simulink model "DEF_IEEE14_case1_phi"  (R2022b)
settings: Solver=FixedStepAuto  StartTime=0  StopTime=10  FixedStep=Ts  RelTol=1e-3
values from neighbouring files (symbols this model uses):
  freq_sel = imag(Mode_Hz)    [Mode_Right_Eig.m]
  Mode_Rad = D(ModeSel, ModeSel)    [Mode_Right_Eig.m]
undefined symbols (not defined in the file or in its folder): ApparatusDiscreDamping, ApparatusPara, ApparatusPowerFlow, ApparatusType, Fbase, OtherInputs, Sbase, Ts, Vbase, Wbase, x_e, Ybase, Zbase
libraries: spsGroundLib x22, SimplusGT x22, spsThreePhaseSeriesRLCBranchLib x20, eeGeneralControl x18, spsThreePhaseParallelRLCBranchLib x14, spsPLLLib x4, spsThreePhaseTransformerTwoWindingsLib x3, spsFourierLib x2, spspowerguiLib x1
settings Model: Creator=y_zhu  LastModifiedBy=y_zhu

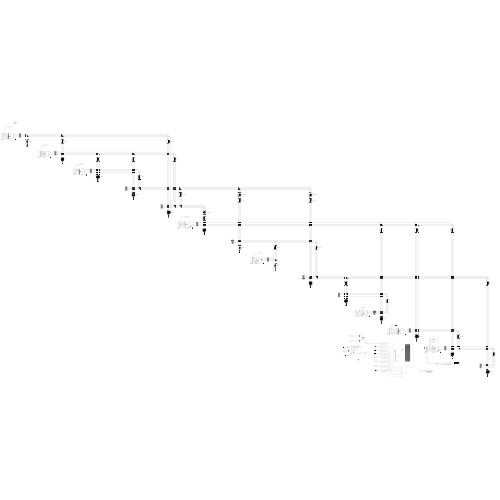
[thumbnail: Simulink's stored preview of the top-level diagram]
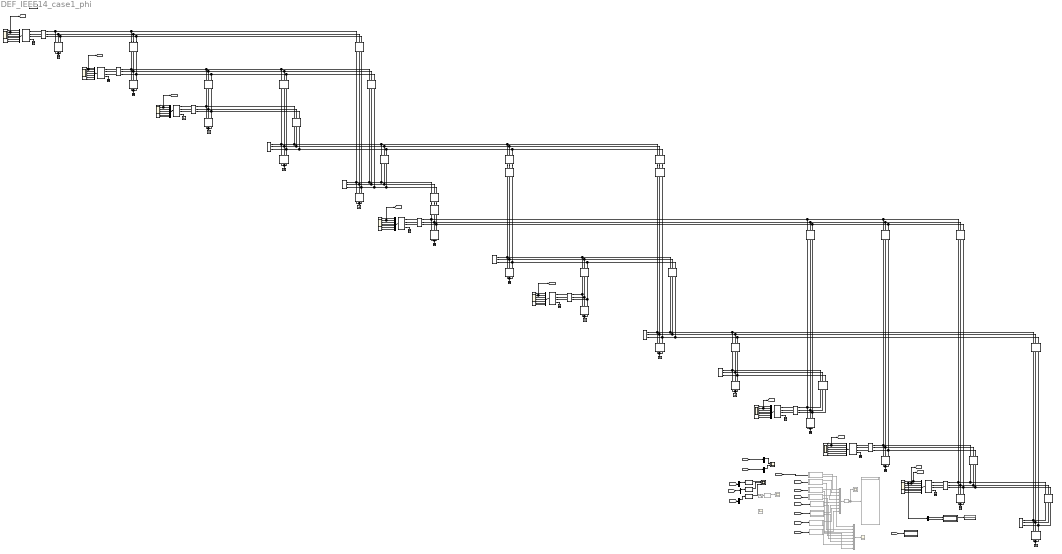
== system DEF_IEEE14_case1_phi ==
  Abs1 : Abs  Commented=on  SaturateOnIntegerOverflow=off
  B-GND{1,4,8,10,14,16,20,23..24,27,29..30,32,34} (14 alike) : spsGroundLib/Ground  LConnTagsString=a
  Branch1-1 : spsThreePhaseParallelRLCBranchLib/Three-Phase Parallel RLC Branch  LConnTagsString=A|B|C  RConnTagsString=A|B|C  BranchType=C  Resistance=(Inf)*Zbase  Inductance=(Inf)*Zbase/Wbase  Capacitance=(0.051)*Ybase/Wbase  Measurements=None
  Branch1-2 : spsThreePhaseSeriesRLCBranchLib/Three-Phase Series RLC Branch  LConnTagsString=A|B|C  RConnTagsString=A|B|C  BranchType=RL  Resistance=(0.01938)*Zbase  Inductance=(0.05917)*Zbase/Wbase  Capacitance=1e-6  Measurements=None
  Branch1-5 : spsThreePhaseSeriesRLCBranchLib/Three-Phase Series RLC Branch  LConnTagsString=A|B|C  RConnTagsString=A|B|C  BranchType=RL  Resistance=(0.05403)*Zbase  Inductance=(0.22304)*Zbase/Wbase  Capacitance=1e-6  Measurements=None
  Branch10-10 : spsThreePhaseParallelRLCBranchLib/Three-Phase Parallel RLC Branch  LConnTagsString=A|B|C  RConnTagsString=A|B|C  BranchType=RLC  Resistance=(12.2907)*Zbase  Inductance=(19.0718)*Zbase/Wbase  Capacitance=(1e-07)*Ybase/Wbase  Measurements=None
  Branch10-11 : spsThreePhaseSeriesRLCBranchLib/Three-Phase Series RLC Branch  LConnTagsString=A|B|C  RConnTagsString=A|B|C  BranchType=RL  Resistance=(0.08205)*Zbase  Inductance=(0.19207)*Zbase/Wbase  Capacitance=1e-6  Measurements=None
  Branch11-11 : spsThreePhaseParallelRLCBranchLib/Three-Phase Parallel RLC Branch  LConnTagsString=A|B|C  RConnTagsString=A|B|C  BranchType=RLC  Resistance=(10.675)*Zbase  Inductance=(62.2711)*Zbase/Wbase  Capacitance=(1e-07)*Ybase/Wbase  Measurements=None
  Branch12-12 : spsThreePhaseParallelRLCBranchLib/Three-Phase Parallel RLC Branch  LConnTagsString=A|B|C  RConnTagsString=A|B|C  BranchType=RLC  Resistance=(6.03)*Zbase  Inductance=(68.9685)*Zbase/Wbase  Capacitance=(1e-07)*Ybase/Wbase  Measurements=None
  Branch12-13 : spsThreePhaseSeriesRLCBranchLib/Three-Phase Series RLC Branch  LConnTagsString=A|B|C  RConnTagsString=A|B|C  BranchType=RL  Resistance=(0.22092)*Zbase  Inductance=(0.19988)*Zbase/Wbase  Capacitance=1e-6  Measurements=None
  Branch13-13 : spsThreePhaseParallelRLCBranchLib/Three-Phase Parallel RLC Branch  LConnTagsString=A|B|C  RConnTagsString=A|B|C  BranchType=RLC  Resistance=(2.6813)*Zbase  Inductance=(18.7232)*Zbase/Wbase  Capacitance=(1.5e-07)*Ybase/Wbase  Measurements=None
  Branch13-14 : spsThreePhaseSeriesRLCBranchLib/Three-Phase Series RLC Branch  LConnTagsString=A|B|C  RConnTagsString=A|B|C  BranchType=RL  Resistance=(0.17093)*Zbase  Inductance=(0.34802)*Zbase/Wbase  Capacitance=1e-6  Measurements=None
  Branch14-14 : spsThreePhaseParallelRLCBranchLib/Three-Phase Parallel RLC Branch  LConnTagsString=A|B|C  RConnTagsString=A|B|C  BranchType=RLC  Resistance=(7.1477)*Zbase  Inductance=(21.3001)*Zbase/Wbase  Capacitance=(1e-07)*Ybase/Wbase  Measurements=None
  Branch2-2 : spsThreePhaseParallelRLCBranchLib/Three-Phase Parallel RLC Branch  LConnTagsString=A|B|C  RConnTagsString=A|B|C  BranchType=RLC  Resistance=(5.0324)*Zbase  Inductance=(8.5986)*Zbase/Wbase  Capacitance=(0.0826)*Ybase/Wbase  Measurements=None
  Branch2-3 : spsThreePhaseSeriesRLCBranchLib/Three-Phase Series RLC Branch  LConnTagsString=A|B|C  RConnTagsString=A|B|C  BranchType=RL  Resistance=(0.04699)*Zbase  Inductance=(0.19797)*Zbase/Wbase  Capacitance=1e-6  Measurements=None
  Branch2-4 : spsThreePhaseSeriesRLCBranchLib/Three-Phase Series RLC Branch  LConnTagsString=A|B|C  RConnTagsString=A|B|C  BranchType=RL  Resistance=(0.05811)*Zbase  Inductance=(0.17632)*Zbase/Wbase  Capacitance=1e-6  Measurements=None
  Branch2-5 : spsThreePhaseSeriesRLCBranchLib/Three-Phase Series RLC Branch  LConnTagsString=A|B|C  RConnTagsString=A|B|C  BranchType=RL  Resistance=(0.05695)*Zbase  Inductance=(0.17388)*Zbase/Wbase  Capacitance=1e-6  Measurements=None
  Branch3-3 : spsThreePhaseParallelRLCBranchLib/Three-Phase Parallel RLC Branch  LConnTagsString=A|B|C  RConnTagsString=A|B|C  BranchType=RLC  Resistance=(1.0829)*Zbase  Inductance=(5.3689)*Zbase/Wbase  Capacitance=(0.0283)*Ybase/Wbase  Measurements=None
  Branch3-4 : spsThreePhaseSeriesRLCBranchLib/Three-Phase Series RLC Branch  LConnTagsString=A|B|C  RConnTagsString=A|B|C  BranchType=RL  Resistance=(0.06701)*Zbase  Inductance=(0.17103)*Zbase/Wbase  Capacitance=1e-6  Measurements=None
  Branch4-4 : spsThreePhaseParallelRLCBranchLib/Three-Phase Parallel RLC Branch  LConnTagsString=A|B|C  RConnTagsString=A|B|C  BranchType=RC  Resistance=(2.1566)*Zbase  Inductance=(Inf)*Zbase/Wbase  Capacitance=(0.061233)*Ybase/Wbase  Measurements=None
  Branch4-5 : spsThreePhaseSeriesRLCBranchLib/Three-Phase Series RLC Branch  LConnTagsString=A|B|C  RConnTagsString=A|B|C  BranchType=RL  Resistance=(0.01335)*Zbase  Inductance=(0.04211)*Zbase/Wbase  Capacitance=1e-6  Measurements=None
  Branch4-7 : spsThreePhaseSeriesRLCBranchLib/Three-Phase Series RLC Branch  LConnTagsString=A|B|C  RConnTagsString=A|B|C  BranchType=RL  Resistance=(1e-07)*Zbase  Inductance=(0.20912)*Zbase/Wbase  Capacitance=1e-6  Measurements=None
  Branch4-9 : spsThreePhaseSeriesRLCBranchLib/Three-Phase Series RLC Branch  LConnTagsString=A|B|C  RConnTagsString=A|B|C  BranchType=RL  Resistance=(1e-07)*Zbase  Inductance=(0.55618)*Zbase/Wbase  Capacitance=1e-6  Measurements=None
  Branch5-5 : spsThreePhaseParallelRLCBranchLib/Three-Phase Parallel RLC Branch  LConnTagsString=A|B|C  RConnTagsString=A|B|C  BranchType=RLC  Resistance=(13.5986)*Zbase  Inductance=(64.5935)*Zbase/Wbase  Capacitance=(0.0419)*Ybase/Wbase  Measurements=None
  Branch5-6 : spsThreePhaseSeriesRLCBranchLib/Three-Phase Series RLC Branch  LConnTagsString=A|B|C  RConnTagsString=A|B|C  BranchType=RL  Resistance=(1e-07)*Zbase  Inductance=(0.25202)*Zbase/Wbase  Capacitance=1e-6  Measurements=None
  Branch6-11 : spsThreePhaseSeriesRLCBranchLib/Three-Phase Series RLC Branch  LConnTagsString=A|B|C  RConnTagsString=A|B|C  BranchType=RL  Resistance=(0.09498)*Zbase  Inductance=(0.1989)*Zbase/Wbase  Capacitance=1e-6  Measurements=None
  Branch6-12 : spsThreePhaseSeriesRLCBranchLib/Three-Phase Series RLC Branch  LConnTagsString=A|B|C  RConnTagsString=A|B|C  BranchType=RL  Resistance=(0.12291)*Zbase  Inductance=(0.25581)*Zbase/Wbase  Capacitance=1e-6  Measurements=None
  Branch6-13 : spsThreePhaseSeriesRLCBranchLib/Three-Phase Series RLC Branch  LConnTagsString=A|B|C  RConnTagsString=A|B|C  BranchType=RL  Resistance=(0.06615)*Zbase  Inductance=(0.13027)*Zbase/Wbase  Capacitance=1e-6  Measurements=None
  Branch6-6 : spsThreePhaseParallelRLCBranchLib/Three-Phase Parallel RLC Branch  LConnTagsString=A|B|C  RConnTagsString=A|B|C  BranchType=RLC  Resistance=(10.2223)*Zbase  Inductance=(15.2653)*Zbase/Wbase  Capacitance=(2e-07)*Ybase/Wbase  Measurements=None
  Branch7-7 : spsThreePhaseParallelRLCBranchLib/Three-Phase Parallel RLC Branch  LConnTagsString=A|B|C  RConnTagsString=A|B|C  BranchType=C  Resistance=(Inf)*Zbase  Inductance=(Inf)*Zbase/Wbase  Capacitance=(1.5e-07)*Ybase/Wbase  Measurements=None
  Branch7-8 : spsThreePhaseSeriesRLCBranchLib/Three-Phase Series RLC Branch  LConnTagsString=A|B|C  RConnTagsString=A|B|C  BranchType=RL  Resistance=(1e-07)*Zbase  Inductance=(0.17615)*Zbase/Wbase  Capacitance=1e-6  Measurements=None
  Branch7-9 : spsThreePhaseSeriesRLCBranchLib/Three-Phase Series RLC Branch  LConnTagsString=A|B|C  RConnTagsString=A|B|C  BranchType=RL  Resistance=(1e-07)*Zbase  Inductance=(0.11001)*Zbase/Wbase  Capacitance=1e-6  Measurements=None
  Branch8-8 : spsThreePhaseParallelRLCBranchLib/Three-Phase Parallel RLC Branch  LConnTagsString=A|B|C  RConnTagsString=A|B|C  BranchType=C  Resistance=(Inf)*Zbase  Inductance=(Inf)*Zbase/Wbase  Capacitance=(5e-08)*Ybase/Wbase  Measurements=None
  Branch9-10 : spsThreePhaseSeriesRLCBranchLib/Three-Phase Series RLC Branch  LConnTagsString=A|B|C  RConnTagsString=A|B|C  BranchType=RL  Resistance=(0.03181)*Zbase  Inductance=(0.0845)*Zbase/Wbase  Capacitance=1e-6  Measurements=None
  Branch9-14 : spsThreePhaseSeriesRLCBranchLib/Three-Phase Series RLC Branch  LConnTagsString=A|B|C  RConnTagsString=A|B|C  BranchType=RL  Resistance=(0.12711)*Zbase  Inductance=(0.27038)*Zbase/Wbase  Capacitance=1e-6  Measurements=None
  Branch9-9 : spsThreePhaseParallelRLCBranchLib/Three-Phase Parallel RLC Branch  LConnTagsString=A|B|C  RConnTagsString=A|B|C  BranchType=RLC  Resistance=(3.7813)*Zbase  Inductance=(6.7198)*Zbase/Wbase  Capacitance=(0.19)*Ybase/Wbase  Measurements=None
  Bus Creator : BusCreator  Commented=on  Inputs=8
  Bus{1..14} (14 alike) : SimplusGT/Three-Phase Bus  Vbase=1  Sbase=1
      settings: SourceProductName=Simplus Grid Tool
  D-GND{1..3,6,8,11..13} (8 alike) : spsGroundLib/Ground  LConnTagsString=a
  D-Scope{1..3,6,8,11..13} (8 alike) : Scope  NumInputPorts=7
  DS-Bus{1..3,6,8,11..13} (8 alike) : BusSelector  OutputSignals=v_dq,i_dq,v_abc,i_abc,w,theta,pq
  Demux{,1..5} (6 alike) : Demux  Outputs=2
  Display : Display
  Display1 : Display  Commented=on
  Mux : Mux  Commented=on  Inputs=8
  PLL : spsPLLLib/PLL  Commented=on  Fmin=freq_sel/2  Par_Init=[0, 0.1]  ParK=[2.4, 1.52*10, 0]  TcD=1  MaxRateChangeFreq=1  FilterCutOffFreq=freq_sel  Ts=1/50  AGC=off
      settings: LibrarySourceBlock=sps_lib/Control/PLL
  PLL1 : spsPLLLib/PLL  Fmin=freq_sel/2  Par_Init=[0, freq_sel]  ParK=[18, 100, 1]  TcD=4e-2  MaxRateChangeFreq=1  FilterCutOffFreq=4  Ts=1e-2  AGC=on
      settings: LibrarySourceBlock=sps_lib/Control/PLL
  PLL2 : spsPLLLib/PLL  Fmin=freq_sel/2  Par_Init=[0, freq_sel]  ParK=[18, 100, 1]  TcD=4e-2  MaxRateChangeFreq=1  FilterCutOffFreq=4  Ts=1e-2  AGC=on
      settings: LibrarySourceBlock=sps_lib/Control/PLL
  PLL3 : spsPLLLib/PLL  Fmin=freq_sel/2  Par_Init=[0, freq_sel]  ParK=[18, 100, 1]  TcD=4e-2  MaxRateChangeFreq=1  FilterCutOffFreq=4  Ts=1e-2  AGC=on
      settings: LibrarySourceBlock=sps_lib/Control/PLL
  SM1 : SimplusGT/SynchronousMachineFull_Cyp_SMAVRPSSGOV (dq-Frame System Object)  Ts=Ts  Sbase=Sbase  Vbase=Vbase  Wbase=Wbase  ApparatusType=ApparatusType{1}  ApparatusPara=ApparatusPara{1}  PowerFlow=ApparatusPowerFlow{1}  x0=x_e{1}  OtherInputs=OtherInputs{1}  DiscreMethod=Hybrid Trapezoidal  EnableInsideModification=off  DiscreDampingFlag=on  DiscreDampingValue=ApparatusDiscreDamping{1}  LinearizationTimes=1  DirectFeedthrough=off
      settings: SourceProductName=Simplus Grid Tool
  SM2 : SimplusGT/SynchronousMachineFull_Cyp_SMAVRPSSGOV (dq-Frame System Object)  Ts=Ts  Sbase=Sbase  Vbase=Vbase  Wbase=Wbase  ApparatusType=ApparatusType{2}  ApparatusPara=ApparatusPara{2}  PowerFlow=ApparatusPowerFlow{2}  x0=x_e{2}  OtherInputs=OtherInputs{2}  DiscreMethod=Hybrid Trapezoidal  EnableInsideModification=off  DiscreDampingFlag=on  DiscreDampingValue=ApparatusDiscreDamping{2}  LinearizationTimes=1  DirectFeedthrough=off
      settings: SourceProductName=Simplus Grid Tool
  SM3 : SimplusGT/SynchronousMachineFull_Cyp_SMAVR (dq-Frame System Object)  Ts=Ts  Sbase=Sbase  Vbase=Vbase  Wbase=Wbase  ApparatusType=ApparatusType{3}  ApparatusPara=ApparatusPara{3}  PowerFlow=ApparatusPowerFlow{3}  x0=x_e{3}  OtherInputs=OtherInputs{3}  DiscreMethod=Hybrid Trapezoidal  EnableInsideModification=off  DiscreDampingFlag=on  DiscreDampingValue=ApparatusDiscreDamping{3}  LinearizationTimes=1  DirectFeedthrough=off
      settings: SourceProductName=Simplus Grid Tool
  SM6 : SimplusGT/SynchronousMachineFull_Cyp_SMAVR (dq-Frame System Object)  Ts=Ts  Sbase=Sbase  Vbase=Vbase  Wbase=Wbase  ApparatusType=ApparatusType{6}  ApparatusPara=ApparatusPara{6}  PowerFlow=ApparatusPowerFlow{6}  x0=x_e{6}  OtherInputs=OtherInputs{6}  DiscreMethod=Hybrid Trapezoidal  EnableInsideModification=off  DiscreDampingFlag=on  DiscreDampingValue=ApparatusDiscreDamping{6}  LinearizationTimes=1  DirectFeedthrough=off
      settings: SourceProductName=Simplus Grid Tool
  SM8 : SimplusGT/SynchronousMachineFull_Cyp_SMAVR (dq-Frame System Object)  Ts=Ts  Sbase=Sbase  Vbase=Vbase  Wbase=Wbase  ApparatusType=ApparatusType{8}  ApparatusPara=ApparatusPara{8}  PowerFlow=ApparatusPowerFlow{8}  x0=x_e{8}  OtherInputs=OtherInputs{8}  DiscreMethod=Hybrid Trapezoidal  EnableInsideModification=off  DiscreDampingFlag=on  DiscreDampingValue=ApparatusDiscreDamping{8}  LinearizationTimes=1  DirectFeedthrough=off
      settings: SourceProductName=Simplus Grid Tool
  SSO_analysis1 : Subsystem  Commented=on
  SSO_analysis2 : Subsystem  Commented=on
  SSO_analysis3 : Subsystem  Commented=on
  SSO_analysis4 : Subsystem  Commented=on
  SSO_analysis5 : Subsystem  Commented=on
  SSO_analysis6 : Subsystem  Commented=on
  SSO_analysis7 : Subsystem  Commented=on
  SSO_analysis8 : Subsystem  Commented=on
  SSO_analysis9 : Subsystem
  Scope : Scope  NumInputPorts=2
  Scope{1..3,5} (4 alike) : Scope  Commented=on
  Scope4 : Scope  NumInputPorts=3
  Sine Wave : Sin  Commented=on  Frequency=freq_sel*2*pi  SampleTime=0
  Subsystem : Subsystem
  Transformer4-7 : spsThreePhaseTransformerTwoWindingsLib/Three-Phase Transformer (Two Windings)  Winding1Connection=Yg  Winding2Connection=Yg  CoreType=Three single-phase transformers  SetSaturation=off  Hysteresis=off  DataFile='hysteresis'  SetInitialFlux=off  Measurements=None  UNITS=pu  NominalPower=[Sbase, Fbase]  Winding1=[0.978*Vbase, 0, 0]  Winding2=[Vbase, 0, 0]  Rm=1e4  Lm=1e4  L0=0.5  Saturation=[ 0,0 ; 0.0024,1.2 ; 1.0,1.52 ]  InitialFluxes=[ 0.8 , -0.8 , 0.7 ]  BreakLoop=off  DiscreteSolver=Trapezoidal iterative  DataType=off  TransfoNumber=1
  Transformer4-9 : spsThreePhaseTransformerTwoWindingsLib/Three-Phase Transformer (Two Windings)  Winding1Connection=Yg  Winding2Connection=Yg  CoreType=Three single-phase transformers  SetSaturation=off  Hysteresis=off  DataFile='hysteresis'  SetInitialFlux=off  Measurements=None  UNITS=pu  NominalPower=[Sbase, Fbase]  Winding1=[0.969*Vbase, 0, 0]  Winding2=[Vbase, 0, 0]  Rm=1e4  Lm=1e4  L0=0.5  Saturation=[ 0,0 ; 0.0024,1.2 ; 1.0,1.52 ]  InitialFluxes=[ 0.8 , -0.8 , 0.7 ]  BreakLoop=off  DiscreteSolver=Trapezoidal iterative  DataType=off  TransfoNumber=1
  Transformer5-6 : spsThreePhaseTransformerTwoWindingsLib/Three-Phase Transformer (Two Windings)  Winding1Connection=Yg  Winding2Connection=Yg  CoreType=Three single-phase transformers  SetSaturation=off  Hysteresis=off  DataFile='hysteresis'  SetInitialFlux=off  Measurements=None  UNITS=pu  NominalPower=[Sbase, Fbase]  Winding1=[0.932*Vbase, 0, 0]  Winding2=[Vbase, 0, 0]  Rm=1e4  Lm=1e4  L0=0.5  Saturation=[ 0,0 ; 0.0024,1.2 ; 1.0,1.52 ]  InitialFluxes=[ 0.8 , -0.8 , 0.7 ]  BreakLoop=off  DiscreteSolver=Trapezoidal iterative  DataType=off  TransfoNumber=1
  VSI-PLL11 : SimplusGT/Grid-Following Voltage-Source Inverter (dq-Frame System Object)  Ts=Ts  Sbase=Sbase  Vbase=Vbase  Wbase=Wbase  ApparatusType=ApparatusType{11}  ApparatusPara=ApparatusPara{11}  PowerFlow=ApparatusPowerFlow{11}  x0=x_e{11}  OtherInputs=OtherInputs{11}  DiscreMethod=Hybrid Trapezoidal  EnableInsideModification=off  DiscreDampingFlag=on  DiscreDampingValue=ApparatusDiscreDamping{11}  LinearizationTimes=1  DirectFeedthrough=off
      settings: SourceProductName=Simplus Grid Tool
  VSI-PLL12 : SimplusGT/Grid-Following Voltage-Source Inverter (dq-Frame System Object)  Ts=Ts  Sbase=Sbase  Vbase=Vbase  Wbase=Wbase  ApparatusType=ApparatusType{12}  ApparatusPara=ApparatusPara{12}  PowerFlow=ApparatusPowerFlow{12}  x0=x_e{12}  OtherInputs=OtherInputs{12}  DiscreMethod=Hybrid Trapezoidal  EnableInsideModification=off  DiscreDampingFlag=on  DiscreDampingValue=ApparatusDiscreDamping{12}  LinearizationTimes=1  DirectFeedthrough=off
      settings: SourceProductName=Simplus Grid Tool
  VSI-PLL13 : SimplusGT/Grid-Following Voltage-Source Inverter (dq-Frame System Object)  Ts=Ts  Sbase=Sbase  Vbase=Vbase  Wbase=Wbase  ApparatusType=ApparatusType{13}  ApparatusPara=ApparatusPara{13}  PowerFlow=ApparatusPowerFlow{13}  x0=x_e{13}  OtherInputs=OtherInputs{13}  DiscreMethod=Hybrid Trapezoidal  EnableInsideModification=off  DiscreDampingFlag=on  DiscreDampingValue=ApparatusDiscreDamping{13}  LinearizationTimes=1  DirectFeedthrough=off
      settings: SourceProductName=Simplus Grid Tool
  powergui : spspowerguiLib/powergui  Priority=1  SimulationMode=Discrete  SampleTime=Ts  frequency=60  Iterations=50  frequencyindice=0  Pbase=100e6  ErrMax=1e-4  UnitsV=kV  UnitsW=MW  buscounter=0  FunctionMessages=off  echomessages=off  EnableUseOfTLC=off  CurrentSourceSwitches=off  DisableSnubberDevices=off  DisableRonSwitches=off  DisableVfSwitches=off  DisplayEquations=off  AutomaticDiscreteSolvers=off  SolverType=Tustin/Backward Euler (TBE)  Interpol=off  ExternalGateDelay=off  methode=off  Ts=100  x0status=blocks  SPID=on  SwTol=0  HookPort=off  NonlinearTolerance=1e-4  nMaxIteration=100  ContinueOnMaxIteration=off  RestoreLinks=warning  ResistiveCurrentMeasurement=off  Frange=[0:2:500]  Ylog=off  Xlog=on  ShowGrid=off  save=off  variable=ZData  structure=0  ZoomFFT=off  StartTime=0.0  cycles=1  DisplayStyle=1  fundamental=60  FreqAxis=off  MaxFrequency=1000  frequencyindicesteady=1  RmsSteady=1  display=off
  wires:
  SM1/1 -> DS-Bus1/1
  DS-Bus1/1 -> D-Scope1/1  "<v_dq>"
  DS-Bus1/3 -> D-Scope1/3  "<v_abc>"
  DS-Bus1/4 -> D-Scope1/4  "<i_abc>"
  DS-Bus1/5 -> D-Scope1/5  "<w>"
  DS-Bus1/6 -> D-Scope1/6  "<theta>"
  DS-Bus1/7 -> D-Scope1/7  "<pq>"
  SM2/1 -> DS-Bus2/1
  DS-Bus2/1 -> D-Scope2/1  "<v_dq>"
  DS-Bus2/3 -> D-Scope2/3  "<v_abc>"
  DS-Bus2/4 -> D-Scope2/4  "<i_abc>"
  DS-Bus2/5 -> D-Scope2/5  "<w>"
  DS-Bus2/6 -> D-Scope2/6  "<theta>"
  DS-Bus2/7 -> D-Scope2/7  "<pq>"
  SM3/1 -> DS-Bus3/1
  DS-Bus3/1 -> D-Scope3/1  "<v_dq>"
  DS-Bus3/3 -> D-Scope3/3  "<v_abc>"
  DS-Bus3/4 -> D-Scope3/4  "<i_abc>"
  DS-Bus3/5 -> D-Scope3/5  "<w>"
  DS-Bus3/6 -> D-Scope3/6  "<theta>"
  DS-Bus3/7 -> D-Scope3/7  "<pq>"
  SM6/1 -> DS-Bus6/1
  DS-Bus6/1 -> D-Scope6/1  "<v_dq>"
  DS-Bus6/2 -> [A6_idq], D-Scope6/2  "<i_dq>"
  DS-Bus6/3 -> D-Scope6/3  "<v_abc>"
  DS-Bus6/4 -> D-Scope6/4  "<i_abc>"
  DS-Bus6/5 -> D-Scope6/5  "<w>"
  DS-Bus6/6 -> D-Scope6/6  "<theta>"
  DS-Bus6/7 -> D-Scope6/7  "<pq>"
  SM8/1 -> DS-Bus8/1
  DS-Bus8/1 -> D-Scope8/1  "<v_dq>"
  DS-Bus8/3 -> D-Scope8/3  "<v_abc>"
  DS-Bus8/4 -> D-Scope8/4  "<i_abc>"
  DS-Bus8/5 -> D-Scope8/5  "<w>"
  DS-Bus8/6 -> D-Scope8/6  "<theta>"
  DS-Bus8/7 -> D-Scope8/7  "<pq>"
  VSI-PLL11/1 -> DS-Bus11/1
  DS-Bus11/1 -> D-Scope11/1  "<v_dq>"
  DS-Bus11/2 -> [A11_idq], D-Scope11/2  "<i_dq>"
  DS-Bus11/3 -> D-Scope11/3  "<v_abc>"
  DS-Bus11/4 -> D-Scope11/4  "<i_abc>"
  DS-Bus11/5 -> D-Scope11/5  "<w>"
  DS-Bus11/6 -> D-Scope11/6  "<theta>"
  DS-Bus11/7 -> D-Scope11/7  "<pq>"
  VSI-PLL12/1 -> DS-Bus12/1
  DS-Bus12/1 -> D-Scope12/1  "<v_dq>"
  DS-Bus12/2 -> [A12_idq], D-Scope12/2  "<i_dq>"
  DS-Bus12/3 -> D-Scope12/3  "<v_abc>"
  DS-Bus12/4 -> D-Scope12/4  "<i_abc>"
  DS-Bus12/5 -> D-Scope12/5  "<w>"
  DS-Bus12/6 -> D-Scope12/6  "<theta>"
  DS-Bus12/7 -> D-Scope12/7  "<pq>"
  VSI-PLL13/1 -> DS-Bus13/1
  DS-Bus13/2 -> [A13_idq], Demux1/1, D-Scope13/2  "<i_dq>"
  DS-Bus13/3 -> D-Scope13/3  "<v_abc>"
  DS-Bus13/4 -> D-Scope13/4  "<i_abc>"
  DS-Bus13/5 -> D-Scope13/5  "<w>"
  DS-Bus13/6 -> D-Scope13/6  "<theta>"
  DS-Bus13/7 -> D-Scope13/7  "<pq>"
  DS-Bus13/1 -> [A13_vdq], D-Scope13/1  "<v_dq>"
  Demux1/1 -> Subsystem/1(id)
  Subsystem/1(id_sso_mag) -> Display/1
  Demux1/2 -> Subsystem/2(iq)
  Mux/1 -> Abs1/1
  [A6_idq] -> SSO_analysis3/1(idq)
  [A11_idq] -> SSO_analysis6/1(idq)
  [A12_idq] -> SSO_analysis7/1(idq)
  [A13_idq] -> SSO_analysis8/1(idq)
  DS-Bus8/2 -> [A8_idq], D-Scope8/2  "<i_dq>"
  [A8_idq] -> SSO_analysis4/1(idq)
  DS-Bus1/2 -> [A1_idq], D-Scope1/2  "<i_dq>"
  DS-Bus2/2 -> [A2_idq], D-Scope2/2  "<i_dq>"
  [A1_idq] -> SSO_analysis5/1(idq)
  [A2_idq] -> SSO_analysis1/1(idq)
  SSO_analysis5/1(idq_sso_abs) -> Mux/1
  SSO_analysis3/1(idq_sso_abs) -> Mux/4
  SSO_analysis4/1(idq_sso_abs) -> Mux/5
  SSO_analysis6/1(idq_sso_abs) -> Mux/6
  SSO_analysis7/1(idq_sso_abs) -> Mux/7
  SSO_analysis8/1(idq_sso_abs) -> Mux/8
  DS-Bus3/2 -> [A3_idq], D-Scope3/2  "<i_dq>"
  [A3_idq] -> SSO_analysis2/1(idq)
  Abs1/1 -> Scope2/1, Display1/1
  SSO_analysis2/1(idq_sso_abs) -> Mux/3
  SSO_analysis1/1(idq_sso_abs) -> Mux/2
  SSO_analysis5/2(idq_sso_abs_sum) -> Bus Creator/1  "A1"
  SSO_analysis1/2(idq_sso_abs_sum) -> Bus Creator/2  "A2"
  SSO_analysis2/2(idq_sso_abs_sum) -> Bus Creator/3  "A3"
  SSO_analysis3/2(idq_sso_abs_sum) -> Bus Creator/4  "A6"
  SSO_analysis4/2(idq_sso_abs_sum) -> Bus Creator/5  "A8"
  SSO_analysis6/2(idq_sso_abs_sum) -> Bus Creator/6  "A11"
  SSO_analysis7/2(idq_sso_abs_sum) -> Bus Creator/7  "A12"
  SSO_analysis8/2(idq_sso_abs_sum) -> Bus Creator/8  "A13"
  Bus Creator/1 -> Scope1/1
  [A13_vdq] -> SSO_analysis9/1(idq)
  [A6_idq] -> Demux/1
  [A12_idq] -> Demux2/1
  Demux/1 -> Scope/1
  Demux2/1 -> Scope/2
  [A6_idq] -> Demux3/1
  [A13_idq] -> Demux4/1
  Sine Wave/1 -> PLL/1
  PLL/1 -> Scope3/1
  Demux3/1 -> PLL1/1
  PLL1/1 -> Scope4/1
  Demux4/1 -> PLL2/1
  PLL2/1 -> Scope4/3
  PLL3/1 -> Scope4/2
  [A12_idq] -> Demux5/1
  Demux5/1 -> PLL3/1
  connections:
  SM1/LConn4 -- D-GND1/LConn1
  SM2/LConn4 -- D-GND2/LConn1
  SM3/LConn4 -- D-GND3/LConn1
  SM6/LConn4 -- D-GND6/LConn1
  SM8/LConn4 -- D-GND8/LConn1
  VSI-PLL11/LConn4 -- D-GND11/LConn1
  VSI-PLL12/LConn4 -- D-GND12/LConn1
  VSI-PLL13/LConn4 -- D-GND13/LConn1
  Branch1-1/RConn1 -- Branch1-1/RConn2 -- Branch1-1/RConn3 -- B-GND1/LConn1
  Branch2-2/RConn1 -- Branch2-2/RConn2 -- Branch2-2/RConn3 -- B-GND4/LConn1
  Branch3-3/RConn1 -- Branch3-3/RConn2 -- Branch3-3/RConn3 -- B-GND8/LConn1
  Branch4-4/RConn1 -- Branch4-4/RConn2 -- Branch4-4/RConn3 -- B-GND10/LConn1
  Branch5-5/RConn1 -- Branch5-5/RConn2 -- Branch5-5/RConn3 -- B-GND14/LConn1
  Branch6-6/RConn1 -- Branch6-6/RConn2 -- Branch6-6/RConn3 -- B-GND16/LConn1
  Branch7-7/RConn1 -- Branch7-7/RConn2 -- Branch7-7/RConn3 -- B-GND20/LConn1
  Branch8-8/RConn1 -- Branch8-8/RConn2 -- Branch8-8/RConn3 -- B-GND23/LConn1
  Branch9-9/RConn1 -- Branch9-9/RConn2 -- Branch9-9/RConn3 -- B-GND24/LConn1
  Branch10-10/RConn1 -- Branch10-10/RConn2 -- Branch10-10/RConn3 -- B-GND27/LConn1
  Branch11-11/RConn1 -- Branch11-11/RConn2 -- Branch11-11/RConn3 -- B-GND29/LConn1
  Branch12-12/RConn1 -- Branch12-12/RConn2 -- Branch12-12/RConn3 -- B-GND30/LConn1
  Branch13-13/RConn1 -- Branch13-13/RConn2 -- Branch13-13/RConn3 -- B-GND32/LConn1
  Branch14-14/RConn1 -- Branch14-14/RConn2 -- Branch14-14/RConn3 -- B-GND34/LConn1
  Branch1-2/RConn1 -- Bus2/RConn1 -- Branch2-2/LConn1 -- Branch2-5/LConn1 -- Branch2-4/LConn1 -- Branch2-3/LConn1
  Branch1-2/RConn2 -- Bus2/RConn2 -- Branch2-2/LConn2 -- Branch2-5/LConn2 -- Branch2-4/LConn2 -- Branch2-3/LConn2
  Branch1-2/RConn3 -- Bus2/RConn3 -- Branch2-2/LConn3 -- Branch2-5/LConn3 -- Branch2-4/LConn3 -- Branch2-3/LConn3
  Branch1-2/LConn1 -- Bus1/RConn1 -- Branch1-1/LConn1 -- Branch1-5/LConn1
  Branch1-2/LConn2 -- Bus1/RConn2 -- Branch1-1/LConn2 -- Branch1-5/LConn2
  Branch1-2/LConn3 -- Bus1/RConn3 -- Branch1-1/LConn3 -- Branch1-5/LConn3
  Branch1-5/RConn1 -- Bus5/RConn1 -- Branch5-5/LConn1 -- Transformer5-6/LConn1 -- Branch4-5/RConn1 -- Branch2-5/RConn1
  Branch1-5/RConn2 -- Bus5/RConn2 -- Branch5-5/LConn2 -- Transformer5-6/LConn2 -- Branch4-5/RConn2 -- Branch2-5/RConn2
  Branch1-5/RConn3 -- Bus5/RConn3 -- Branch5-5/LConn3 -- Transformer5-6/LConn3 -- Branch4-5/RConn3 -- Branch2-5/RConn3
  Branch2-3/RConn1 -- Bus3/RConn1 -- Branch3-3/LConn1 -- Branch3-4/LConn1
  Branch2-3/RConn2 -- Bus3/RConn2 -- Branch3-3/LConn2 -- Branch3-4/LConn2
  Branch2-3/RConn3 -- Bus3/RConn3 -- Branch3-3/LConn3 -- Branch3-4/LConn3
  Branch2-4/RConn1 -- Bus4/RConn1 -- Branch4-4/LConn1 -- Transformer4-9/LConn1 -- Transformer4-7/LConn1 -- Branch4-5/LConn1 -- Branch3-4/RConn1
  Branch2-4/RConn2 -- Bus4/RConn2 -- Branch4-4/LConn2 -- Transformer4-9/LConn2 -- Transformer4-7/LConn2 -- Branch4-5/LConn2 -- Branch3-4/RConn2
  Branch2-4/RConn3 -- Bus4/RConn3 -- Branch4-4/LConn3 -- Transformer4-9/LConn3 -- Transformer4-7/LConn3 -- Branch4-5/LConn3 -- Branch3-4/RConn3
  Branch4-7/RConn1 -- Bus7/RConn1 -- Branch7-7/LConn1 -- Branch7-9/LConn1 -- Branch7-8/LConn1
  Branch4-7/RConn2 -- Bus7/RConn2 -- Branch7-7/LConn2 -- Branch7-9/LConn2 -- Branch7-8/LConn2
  Branch4-7/RConn3 -- Bus7/RConn3 -- Branch7-7/LConn3 -- Branch7-9/LConn3 -- Branch7-8/LConn3
  Transformer4-7/RConn1 -- Branch4-7/LConn1
  Transformer4-7/RConn2 -- Branch4-7/LConn2
  Transformer4-7/RConn3 -- Branch4-7/LConn3
  Branch4-9/RConn1 -- Bus9/RConn1 -- Branch9-9/LConn1 -- Branch9-14/LConn1 -- Branch9-10/LConn1 -- Branch7-9/RConn1
  Branch4-9/RConn2 -- Bus9/RConn2 -- Branch9-9/LConn2 -- Branch9-14/LConn2 -- Branch9-10/LConn2 -- Branch7-9/RConn2
  Branch4-9/RConn3 -- Bus9/RConn3 -- Branch9-9/LConn3 -- Branch9-14/LConn3 -- Branch9-10/LConn3 -- Branch7-9/RConn3
  Transformer4-9/RConn1 -- Branch4-9/LConn1
  Transformer4-9/RConn2 -- Branch4-9/LConn2
  Transformer4-9/RConn3 -- Branch4-9/LConn3
  Branch5-6/RConn1 -- Bus6/RConn1 -- Branch6-6/LConn1 -- Branch6-13/LConn1 -- Branch6-12/LConn1 -- Branch6-11/LConn1
  Branch5-6/RConn2 -- Bus6/RConn2 -- Branch6-6/LConn2 -- Branch6-13/LConn2 -- Branch6-12/LConn2 -- Branch6-11/LConn2
  Branch5-6/RConn3 -- Bus6/RConn3 -- Branch6-6/LConn3 -- Branch6-13/LConn3 -- Branch6-12/LConn3 -- Branch6-11/LConn3
  Transformer5-6/RConn1 -- Branch5-6/LConn1
  Transformer5-6/RConn2 -- Branch5-6/LConn2
  Transformer5-6/RConn3 -- Branch5-6/LConn3
  Branch6-11/RConn1 -- Bus11/RConn1 -- Branch11-11/LConn1 -- Branch10-11/RConn1
  Branch6-11/RConn2 -- Bus11/RConn2 -- Branch11-11/LConn2 -- Branch10-11/RConn2
  Branch6-11/RConn3 -- Bus11/RConn3 -- Branch11-11/LConn3 -- Branch10-11/RConn3
  Branch6-12/RConn1 -- Bus12/RConn1 -- Branch12-12/LConn1 -- Branch12-13/LConn1
  Branch6-12/RConn2 -- Bus12/RConn2 -- Branch12-12/LConn2 -- Branch12-13/LConn2
  Branch6-12/RConn3 -- Bus12/RConn3 -- Branch12-12/LConn3 -- Branch12-13/LConn3
  Branch6-13/RConn1 -- Bus13/RConn1 -- Branch13-13/LConn1 -- Branch13-14/LConn1 -- Branch12-13/RConn1
  Branch6-13/RConn2 -- Bus13/RConn2 -- Branch13-13/LConn2 -- Branch13-14/LConn2 -- Branch12-13/RConn2
  Branch6-13/RConn3 -- Bus13/RConn3 -- Branch13-13/LConn3 -- Branch13-14/LConn3 -- Branch12-13/RConn3
  Branch7-8/RConn1 -- Bus8/RConn1 -- Branch8-8/LConn1
  Branch7-8/RConn2 -- Bus8/RConn2 -- Branch8-8/LConn2
  Branch7-8/RConn3 -- Bus8/RConn3 -- Branch8-8/LConn3
  Branch9-10/RConn1 -- Bus10/RConn1 -- Branch10-10/LConn1 -- Branch10-11/LConn1
  Branch9-10/RConn2 -- Bus10/RConn2 -- Branch10-10/LConn2 -- Branch10-11/LConn2
  Branch9-10/RConn3 -- Bus10/RConn3 -- Branch10-10/LConn3 -- Branch10-11/LConn3
  Branch9-14/RConn1 -- Bus14/RConn1 -- Branch14-14/LConn1 -- Branch13-14/RConn1
  Branch9-14/RConn2 -- Bus14/RConn2 -- Branch14-14/LConn2 -- Branch13-14/RConn2
  Branch9-14/RConn3 -- Bus14/RConn3 -- Branch14-14/LConn3 -- Branch13-14/RConn3
  SM1/LConn1 -- Bus1/LConn1
  SM1/LConn2 -- Bus1/LConn2
  SM1/LConn3 -- Bus1/LConn3
  SM2/LConn1 -- Bus2/LConn1
  SM2/LConn2 -- Bus2/LConn2
  SM2/LConn3 -- Bus2/LConn3
  SM3/LConn1 -- Bus3/LConn1
  SM3/LConn2 -- Bus3/LConn2
  SM3/LConn3 -- Bus3/LConn3
  SM6/LConn1 -- Bus6/LConn1
  SM6/LConn2 -- Bus6/LConn2
  SM6/LConn3 -- Bus6/LConn3
  SM8/LConn1 -- Bus8/LConn1
  SM8/LConn2 -- Bus8/LConn2
  SM8/LConn3 -- Bus8/LConn3
  VSI-PLL11/LConn1 -- Bus11/LConn1
  VSI-PLL11/LConn2 -- Bus11/LConn2
  VSI-PLL11/LConn3 -- Bus11/LConn3
  VSI-PLL12/LConn1 -- Bus12/LConn1
  VSI-PLL12/LConn2 -- Bus12/LConn2
  VSI-PLL12/LConn3 -- Bus12/LConn3
  VSI-PLL13/LConn1 -- Bus13/LConn1
  VSI-PLL13/LConn2 -- Bus13/LConn2
  VSI-PLL13/LConn3 -- Bus13/LConn3

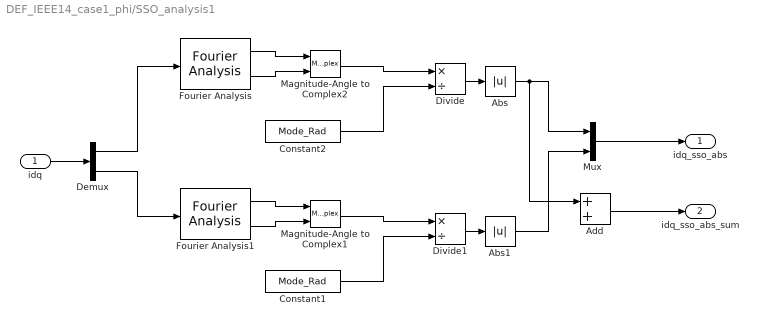
== system DEF_IEEE14_case1_phi/SSO_analysis1 ==
  idq : Inport
  Abs : Abs  SaturateOnIntegerOverflow=off
  Abs1 : Abs  SaturateOnIntegerOverflow=off
  Add : Sum
  Constant1 : Constant  Value=Mode_Rad
  Constant2 : Constant  Value=Mode_Rad
  Demux : Demux  Outputs=2
  Divide : Product  Inputs=*/
  Divide1 : Product  Inputs=*/
  Fourier Analysis : eeGeneralControl/Fourier Analysis  f=freq_sel/3  n=3  M0=0  Ph0=0  BufferSize=8192  Ts=1/50
      settings: LibrarySourceBlock=ee_sl_lib/General Control/Fourier Analysis
  Fourier Analysis1 : eeGeneralControl/Fourier Analysis  f=freq_sel/3  n=3  M0=0  Ph0=0  BufferSize=8192  Ts=1/50
      settings: LibrarySourceBlock=ee_sl_lib/General Control/Fourier Analysis
  Magnitude-Angle to Complex1 : MagnitudeAngleToComplex
  Magnitude-Angle to Complex2 : MagnitudeAngleToComplex
  Mux : Mux  Inputs=2
  idq_sso_abs : Outport
  idq_sso_abs_sum : Outport  Port=2
  wires:
  Constant2/1 -> Divide/2
  idq/1 -> Demux/1
  Demux/1 -> Fourier Analysis/1
  Fourier Analysis/1 -> Magnitude-Angle to Complex2/1
  Fourier Analysis/2 -> Magnitude-Angle to Complex2/2
  Magnitude-Angle to Complex2/1 -> Divide/1
  Mux/1 -> idq_sso_abs/1
  Divide/1 -> Abs/1
  Fourier Analysis1/2 -> Magnitude-Angle to Complex1/2
  Fourier Analysis1/1 -> Magnitude-Angle to Complex1/1
  Magnitude-Angle to Complex1/1 -> Divide1/1
  Constant1/1 -> Divide1/2
  Demux/2 -> Fourier Analysis1/1
  Divide1/1 -> Abs1/1
  Abs/1 -> Add/1, Mux/1
  Abs1/1 -> Mux/2
  Add/1 -> idq_sso_abs_sum/1

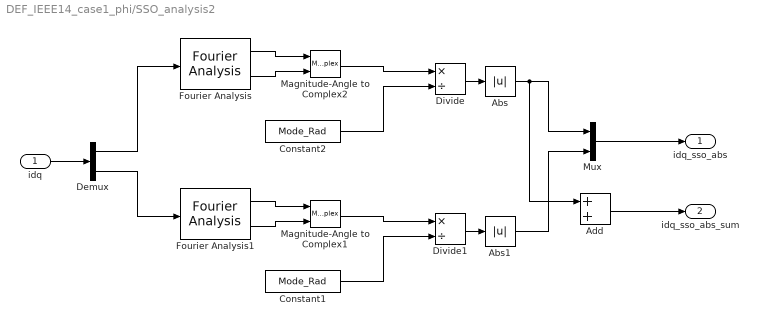
== system DEF_IEEE14_case1_phi/SSO_analysis2 ==
  idq : Inport
  Abs : Abs  SaturateOnIntegerOverflow=off
  Abs1 : Abs  SaturateOnIntegerOverflow=off
  Add : Sum
  Constant1 : Constant  Value=Mode_Rad
  Constant2 : Constant  Value=Mode_Rad
  Demux : Demux  Outputs=2
  Divide : Product  Inputs=*/
  Divide1 : Product  Inputs=*/
  Fourier Analysis : eeGeneralControl/Fourier Analysis  f=freq_sel/3  n=3  M0=0  Ph0=0  BufferSize=8192  Ts=1/50
      settings: LibrarySourceBlock=ee_sl_lib/General Control/Fourier Analysis
  Fourier Analysis1 : eeGeneralControl/Fourier Analysis  f=freq_sel/3  n=3  M0=0  Ph0=0  BufferSize=8192  Ts=1/50
      settings: LibrarySourceBlock=ee_sl_lib/General Control/Fourier Analysis
  Magnitude-Angle to Complex1 : MagnitudeAngleToComplex
  Magnitude-Angle to Complex2 : MagnitudeAngleToComplex
  Mux : Mux  Inputs=2
  idq_sso_abs : Outport
  idq_sso_abs_sum : Outport  Port=2
  wires:
  Constant2/1 -> Divide/2
  idq/1 -> Demux/1
  Demux/1 -> Fourier Analysis/1
  Fourier Analysis/1 -> Magnitude-Angle to Complex2/1
  Fourier Analysis/2 -> Magnitude-Angle to Complex2/2
  Magnitude-Angle to Complex2/1 -> Divide/1
  Mux/1 -> idq_sso_abs/1
  Divide/1 -> Abs/1
  Fourier Analysis1/2 -> Magnitude-Angle to Complex1/2
  Fourier Analysis1/1 -> Magnitude-Angle to Complex1/1
  Magnitude-Angle to Complex1/1 -> Divide1/1
  Constant1/1 -> Divide1/2
  Demux/2 -> Fourier Analysis1/1
  Divide1/1 -> Abs1/1
  Abs/1 -> Add/1, Mux/1
  Abs1/1 -> Mux/2
  Add/1 -> idq_sso_abs_sum/1

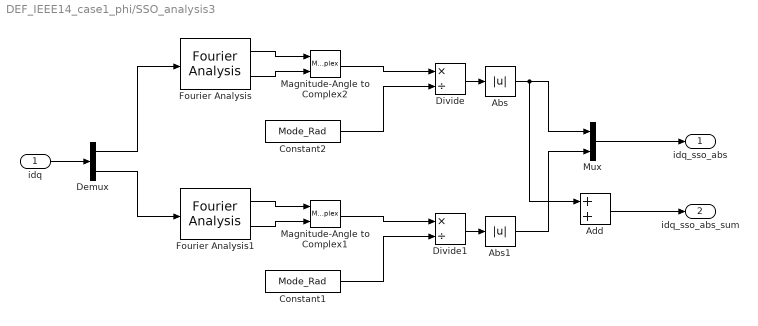
== system DEF_IEEE14_case1_phi/SSO_analysis3 ==
  idq : Inport
  Abs : Abs  SaturateOnIntegerOverflow=off
  Abs1 : Abs  SaturateOnIntegerOverflow=off
  Add : Sum
  Constant1 : Constant  Value=Mode_Rad
  Constant2 : Constant  Value=Mode_Rad
  Demux : Demux  Outputs=2
  Divide : Product  Inputs=*/
  Divide1 : Product  Inputs=*/
  Fourier Analysis : eeGeneralControl/Fourier Analysis  f=freq_sel/3  n=3  M0=0  Ph0=0  BufferSize=8192  Ts=1/50
      settings: LibrarySourceBlock=ee_sl_lib/General Control/Fourier Analysis
  Fourier Analysis1 : eeGeneralControl/Fourier Analysis  f=freq_sel/3  n=3  M0=0  Ph0=0  BufferSize=8192  Ts=1/50
      settings: LibrarySourceBlock=ee_sl_lib/General Control/Fourier Analysis
  Magnitude-Angle to Complex1 : MagnitudeAngleToComplex
  Magnitude-Angle to Complex2 : MagnitudeAngleToComplex
  Mux : Mux  Inputs=2
  idq_sso_abs : Outport
  idq_sso_abs_sum : Outport  Port=2
  wires:
  Constant2/1 -> Divide/2
  idq/1 -> Demux/1
  Demux/1 -> Fourier Analysis/1
  Fourier Analysis/1 -> Magnitude-Angle to Complex2/1
  Fourier Analysis/2 -> Magnitude-Angle to Complex2/2
  Magnitude-Angle to Complex2/1 -> Divide/1
  Mux/1 -> idq_sso_abs/1
  Divide/1 -> Abs/1
  Fourier Analysis1/2 -> Magnitude-Angle to Complex1/2
  Fourier Analysis1/1 -> Magnitude-Angle to Complex1/1
  Magnitude-Angle to Complex1/1 -> Divide1/1
  Constant1/1 -> Divide1/2
  Demux/2 -> Fourier Analysis1/1
  Divide1/1 -> Abs1/1
  Abs/1 -> Add/1, Mux/1
  Abs1/1 -> Mux/2
  Add/1 -> idq_sso_abs_sum/1

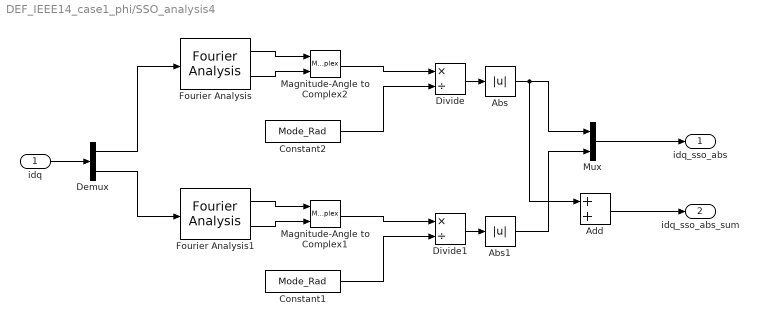
== system DEF_IEEE14_case1_phi/SSO_analysis4 ==
  idq : Inport
  Abs : Abs  SaturateOnIntegerOverflow=off
  Abs1 : Abs  SaturateOnIntegerOverflow=off
  Add : Sum
  Constant1 : Constant  Value=Mode_Rad
  Constant2 : Constant  Value=Mode_Rad
  Demux : Demux  Outputs=2
  Divide : Product  Inputs=*/
  Divide1 : Product  Inputs=*/
  Fourier Analysis : eeGeneralControl/Fourier Analysis  f=freq_sel/3  n=3  M0=0  Ph0=0  BufferSize=8192  Ts=1/50
      settings: LibrarySourceBlock=ee_sl_lib/General Control/Fourier Analysis
  Fourier Analysis1 : eeGeneralControl/Fourier Analysis  f=freq_sel/3  n=3  M0=0  Ph0=0  BufferSize=8192  Ts=1/50
      settings: LibrarySourceBlock=ee_sl_lib/General Control/Fourier Analysis
  Magnitude-Angle to Complex1 : MagnitudeAngleToComplex
  Magnitude-Angle to Complex2 : MagnitudeAngleToComplex
  Mux : Mux  Inputs=2
  idq_sso_abs : Outport
  idq_sso_abs_sum : Outport  Port=2
  wires:
  Constant2/1 -> Divide/2
  idq/1 -> Demux/1
  Demux/1 -> Fourier Analysis/1
  Fourier Analysis/1 -> Magnitude-Angle to Complex2/1
  Fourier Analysis/2 -> Magnitude-Angle to Complex2/2
  Magnitude-Angle to Complex2/1 -> Divide/1
  Mux/1 -> idq_sso_abs/1
  Divide/1 -> Abs/1
  Fourier Analysis1/2 -> Magnitude-Angle to Complex1/2
  Fourier Analysis1/1 -> Magnitude-Angle to Complex1/1
  Magnitude-Angle to Complex1/1 -> Divide1/1
  Constant1/1 -> Divide1/2
  Demux/2 -> Fourier Analysis1/1
  Divide1/1 -> Abs1/1
  Abs/1 -> Add/1, Mux/1
  Abs1/1 -> Mux/2
  Add/1 -> idq_sso_abs_sum/1

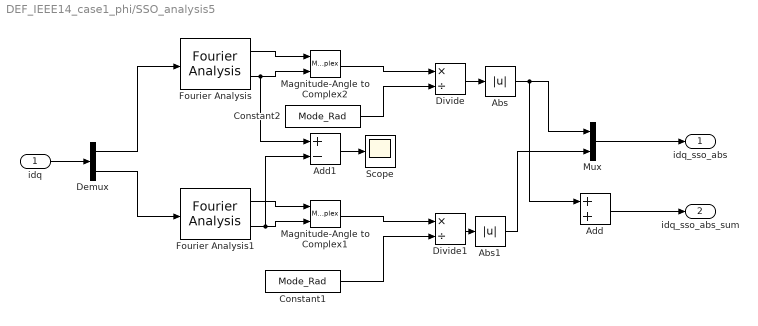
== system DEF_IEEE14_case1_phi/SSO_analysis5 ==
  idq : Inport
  Abs : Abs  SaturateOnIntegerOverflow=off
  Abs1 : Abs  SaturateOnIntegerOverflow=off
  Add : Sum
  Add1 : Sum  Inputs=+-
  Constant1 : Constant  Value=Mode_Rad
  Constant2 : Constant  Value=Mode_Rad
  Demux : Demux  Outputs=2
  Divide : Product  Inputs=*/
  Divide1 : Product  Inputs=*/
  Fourier Analysis : eeGeneralControl/Fourier Analysis  f=freq_sel/3  n=3  M0=0  Ph0=0  BufferSize=8192  Ts=1/50
      settings: LibrarySourceBlock=ee_sl_lib/General Control/Fourier Analysis
  Fourier Analysis1 : eeGeneralControl/Fourier Analysis  f=freq_sel/3  n=3  M0=0  Ph0=0  BufferSize=8192  Ts=1/50
      settings: LibrarySourceBlock=ee_sl_lib/General Control/Fourier Analysis
  Magnitude-Angle to Complex1 : MagnitudeAngleToComplex
  Magnitude-Angle to Complex2 : MagnitudeAngleToComplex
  Mux : Mux  Inputs=2
  Scope : Scope
  idq_sso_abs : Outport
  idq_sso_abs_sum : Outport  Port=2
  wires:
  Constant2/1 -> Divide/2
  idq/1 -> Demux/1
  Demux/1 -> Fourier Analysis/1
  Fourier Analysis/1 -> Magnitude-Angle to Complex2/1
  Fourier Analysis/2 -> Add1/1, Magnitude-Angle to Complex2/2
  Magnitude-Angle to Complex2/1 -> Divide/1
  Mux/1 -> idq_sso_abs/1
  Divide/1 -> Abs/1
  Fourier Analysis1/2 -> Add1/2, Magnitude-Angle to Complex1/2
  Fourier Analysis1/1 -> Magnitude-Angle to Complex1/1
  Magnitude-Angle to Complex1/1 -> Divide1/1
  Constant1/1 -> Divide1/2
  Demux/2 -> Fourier Analysis1/1
  Divide1/1 -> Abs1/1
  Abs/1 -> Add/1, Mux/1
  Abs1/1 -> Mux/2
  Add/1 -> idq_sso_abs_sum/1
  Add1/1 -> Scope/1

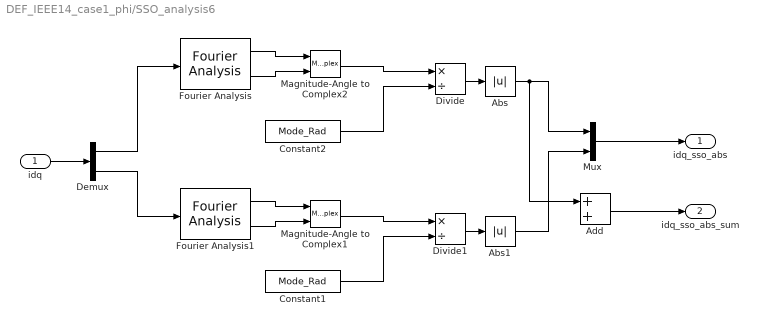
== system DEF_IEEE14_case1_phi/SSO_analysis6 ==
  idq : Inport
  Abs : Abs  SaturateOnIntegerOverflow=off
  Abs1 : Abs  SaturateOnIntegerOverflow=off
  Add : Sum
  Constant1 : Constant  Value=Mode_Rad
  Constant2 : Constant  Value=Mode_Rad
  Demux : Demux  Outputs=2
  Divide : Product  Inputs=*/
  Divide1 : Product  Inputs=*/
  Fourier Analysis : eeGeneralControl/Fourier Analysis  f=freq_sel/3  n=3  M0=0  Ph0=0  BufferSize=8192  Ts=1/50
      settings: LibrarySourceBlock=ee_sl_lib/General Control/Fourier Analysis
  Fourier Analysis1 : eeGeneralControl/Fourier Analysis  f=freq_sel/3  n=3  M0=0  Ph0=0  BufferSize=8192  Ts=1/50
      settings: LibrarySourceBlock=ee_sl_lib/General Control/Fourier Analysis
  Magnitude-Angle to Complex1 : MagnitudeAngleToComplex
  Magnitude-Angle to Complex2 : MagnitudeAngleToComplex
  Mux : Mux  Inputs=2
  idq_sso_abs : Outport
  idq_sso_abs_sum : Outport  Port=2
  wires:
  Constant2/1 -> Divide/2
  idq/1 -> Demux/1
  Demux/1 -> Fourier Analysis/1
  Fourier Analysis/1 -> Magnitude-Angle to Complex2/1
  Fourier Analysis/2 -> Magnitude-Angle to Complex2/2
  Magnitude-Angle to Complex2/1 -> Divide/1
  Mux/1 -> idq_sso_abs/1
  Divide/1 -> Abs/1
  Fourier Analysis1/2 -> Magnitude-Angle to Complex1/2
  Fourier Analysis1/1 -> Magnitude-Angle to Complex1/1
  Magnitude-Angle to Complex1/1 -> Divide1/1
  Constant1/1 -> Divide1/2
  Demux/2 -> Fourier Analysis1/1
  Divide1/1 -> Abs1/1
  Abs/1 -> Add/1, Mux/1
  Abs1/1 -> Mux/2
  Add/1 -> idq_sso_abs_sum/1

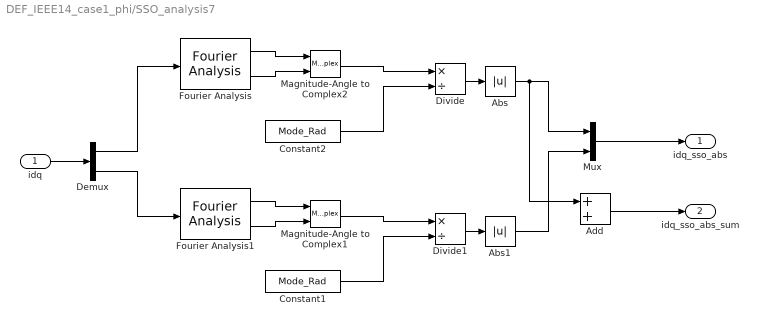
== system DEF_IEEE14_case1_phi/SSO_analysis7 ==
  idq : Inport
  Abs : Abs  SaturateOnIntegerOverflow=off
  Abs1 : Abs  SaturateOnIntegerOverflow=off
  Add : Sum
  Constant1 : Constant  Value=Mode_Rad
  Constant2 : Constant  Value=Mode_Rad
  Demux : Demux  Outputs=2
  Divide : Product  Inputs=*/
  Divide1 : Product  Inputs=*/
  Fourier Analysis : eeGeneralControl/Fourier Analysis  f=freq_sel/3  n=3  M0=0  Ph0=0  BufferSize=8192  Ts=1/50
      settings: LibrarySourceBlock=ee_sl_lib/General Control/Fourier Analysis
  Fourier Analysis1 : eeGeneralControl/Fourier Analysis  f=freq_sel/3  n=3  M0=0  Ph0=0  BufferSize=8192  Ts=1/50
      settings: LibrarySourceBlock=ee_sl_lib/General Control/Fourier Analysis
  Magnitude-Angle to Complex1 : MagnitudeAngleToComplex
  Magnitude-Angle to Complex2 : MagnitudeAngleToComplex
  Mux : Mux  Inputs=2
  idq_sso_abs : Outport
  idq_sso_abs_sum : Outport  Port=2
  wires:
  Constant2/1 -> Divide/2
  idq/1 -> Demux/1
  Demux/1 -> Fourier Analysis/1
  Fourier Analysis/1 -> Magnitude-Angle to Complex2/1
  Fourier Analysis/2 -> Magnitude-Angle to Complex2/2
  Magnitude-Angle to Complex2/1 -> Divide/1
  Mux/1 -> idq_sso_abs/1
  Divide/1 -> Abs/1
  Fourier Analysis1/2 -> Magnitude-Angle to Complex1/2
  Fourier Analysis1/1 -> Magnitude-Angle to Complex1/1
  Magnitude-Angle to Complex1/1 -> Divide1/1
  Constant1/1 -> Divide1/2
  Demux/2 -> Fourier Analysis1/1
  Divide1/1 -> Abs1/1
  Abs/1 -> Add/1, Mux/1
  Abs1/1 -> Mux/2
  Add/1 -> idq_sso_abs_sum/1

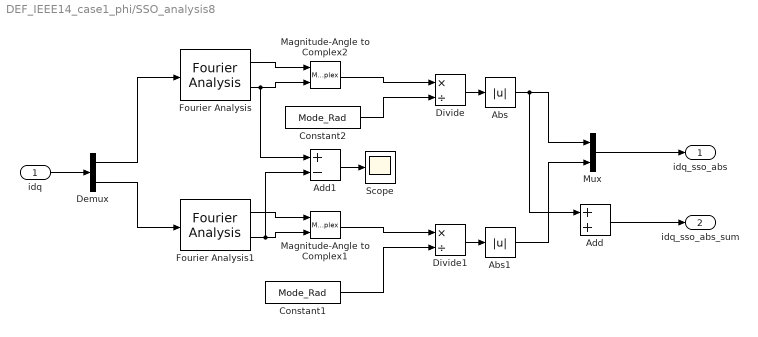
== system DEF_IEEE14_case1_phi/SSO_analysis8 ==
  idq : Inport
  Abs : Abs  SaturateOnIntegerOverflow=off
  Abs1 : Abs  SaturateOnIntegerOverflow=off
  Add : Sum
  Add1 : Sum  Inputs=+-
  Constant1 : Constant  Value=Mode_Rad
  Constant2 : Constant  Value=Mode_Rad
  Demux : Demux  Outputs=2
  Divide : Product  Inputs=*/
  Divide1 : Product  Inputs=*/
  Fourier Analysis : eeGeneralControl/Fourier Analysis  f=freq_sel/3  n=3  M0=0  Ph0=0  BufferSize=8192  Ts=1/50
      settings: LibrarySourceBlock=ee_sl_lib/General Control/Fourier Analysis
  Fourier Analysis1 : eeGeneralControl/Fourier Analysis  f=freq_sel/3  n=3  M0=0  Ph0=0  BufferSize=8192  Ts=1/50
      settings: LibrarySourceBlock=ee_sl_lib/General Control/Fourier Analysis
  Magnitude-Angle to Complex1 : MagnitudeAngleToComplex
  Magnitude-Angle to Complex2 : MagnitudeAngleToComplex
  Mux : Mux  Inputs=2
  Scope : Scope
  idq_sso_abs : Outport
  idq_sso_abs_sum : Outport  Port=2
  wires:
  Constant2/1 -> Divide/2
  idq/1 -> Demux/1
  Demux/1 -> Fourier Analysis/1
  Fourier Analysis/1 -> Magnitude-Angle to Complex2/1
  Magnitude-Angle to Complex2/1 -> Divide/1
  Mux/1 -> idq_sso_abs/1
  Divide/1 -> Abs/1
  Fourier Analysis1/1 -> Magnitude-Angle to Complex1/1
  Magnitude-Angle to Complex1/1 -> Divide1/1
  Constant1/1 -> Divide1/2
  Demux/2 -> Fourier Analysis1/1
  Divide1/1 -> Abs1/1
  Abs/1 -> Add/1, Mux/1
  Abs1/1 -> Mux/2
  Add/1 -> idq_sso_abs_sum/1
  Add1/1 -> Scope/1
  Fourier Analysis/2 -> Add1/1, Magnitude-Angle to Complex2/2
  Fourier Analysis1/2 -> Add1/2, Magnitude-Angle to Complex1/2

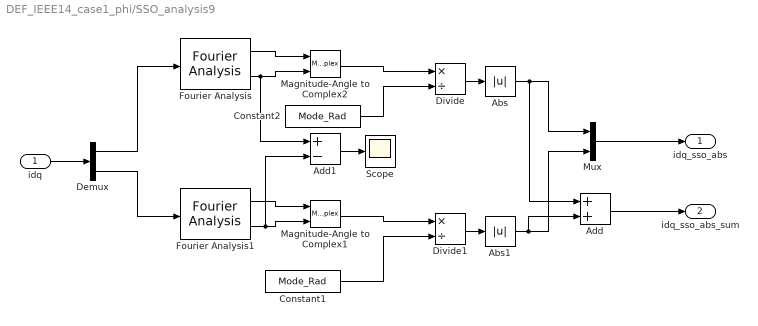
== system DEF_IEEE14_case1_phi/SSO_analysis9 ==
  idq : Inport
  Abs : Abs  SaturateOnIntegerOverflow=off
  Abs1 : Abs  SaturateOnIntegerOverflow=off
  Add : Sum
  Add1 : Sum  Inputs=+-
  Constant1 : Constant  Value=Mode_Rad
  Constant2 : Constant  Value=Mode_Rad
  Demux : Demux  Outputs=2
  Divide : Product  Inputs=*/
  Divide1 : Product  Inputs=*/
  Fourier Analysis : eeGeneralControl/Fourier Analysis  f=freq_sel/3  n=3  M0=0  Ph0=0  BufferSize=8192  Ts=1/50
      settings: LibrarySourceBlock=ee_sl_lib/General Control/Fourier Analysis
  Fourier Analysis1 : eeGeneralControl/Fourier Analysis  f=freq_sel/3  n=3  M0=0  Ph0=0  BufferSize=8192  Ts=1/50
      settings: LibrarySourceBlock=ee_sl_lib/General Control/Fourier Analysis
  Magnitude-Angle to Complex1 : MagnitudeAngleToComplex
  Magnitude-Angle to Complex2 : MagnitudeAngleToComplex
  Mux : Mux  Inputs=2
  Scope : Scope
  idq_sso_abs : Outport
  idq_sso_abs_sum : Outport  Port=2
  wires:
  Constant2/1 -> Divide/2
  idq/1 -> Demux/1
  Demux/1 -> Fourier Analysis/1
  Fourier Analysis/1 -> Magnitude-Angle to Complex2/1
  Fourier Analysis/2 -> Add1/1, Magnitude-Angle to Complex2/2
  Magnitude-Angle to Complex2/1 -> Divide/1
  Mux/1 -> idq_sso_abs/1
  Divide/1 -> Abs/1
  Fourier Analysis1/2 -> Add1/2, Magnitude-Angle to Complex1/2
  Fourier Analysis1/1 -> Magnitude-Angle to Complex1/1
  Magnitude-Angle to Complex1/1 -> Divide1/1
  Constant1/1 -> Divide1/2
  Demux/2 -> Fourier Analysis1/1
  Divide1/1 -> Abs1/1
  Abs/1 -> Add/1, Mux/1
  Abs1/1 -> Add/2, Mux/2
  Add/1 -> idq_sso_abs_sum/1
  Add1/1 -> Scope/1

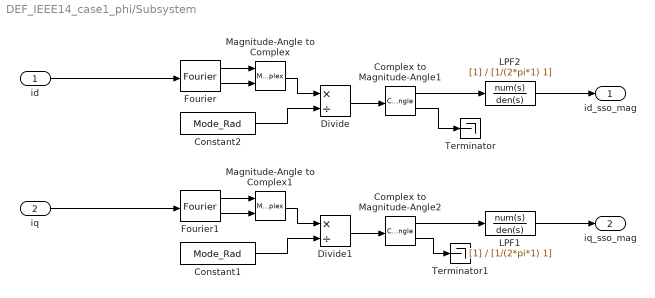
== system DEF_IEEE14_case1_phi/Subsystem ==
  id : Inport
  iq : Inport  Port=2
  Complex to Magnitude-Angle1 : ComplexToMagnitudeAngle
  Complex to Magnitude-Angle2 : ComplexToMagnitudeAngle
  Constant1 : Constant  Value=Mode_Rad
  Constant2 : Constant  Value=Mode_Rad
  Divide : Product  Inputs=*/
  Divide1 : Product  Inputs=*/
  Fourier : spsFourierLib/Fourier  Freq=freq_sel  n=1  InInit=[0, 0]  Ts=0
  Fourier1 : spsFourierLib/Fourier  Freq=freq_sel  n=1  InInit=[0, 0]  Ts=0
  LPF1 : TransferFcn  Denominator=[1/(2*pi*1) 1]
  LPF2 : TransferFcn  Denominator=[1/(2*pi*1) 1]
  Magnitude-Angle to Complex : MagnitudeAngleToComplex
  Magnitude-Angle to Complex1 : MagnitudeAngleToComplex
  Terminator : Terminator
  Terminator1 : Terminator
  id_sso_mag : Outport
  iq_sso_mag : Outport  Port=2
  wires:
  Complex to Magnitude-Angle1/2 -> Terminator/1
  Fourier/1 -> Magnitude-Angle to Complex/1
  Constant2/1 -> Divide/2
  Magnitude-Angle to Complex/1 -> Divide/1
  Divide/1 -> Complex to Magnitude-Angle1/1
  Complex to Magnitude-Angle1/1 -> LPF2/1
  Fourier/2 -> Magnitude-Angle to Complex/2
  LPF2/1 -> id_sso_mag/1
  id/1 -> Fourier/1
  Divide1/1 -> Complex to Magnitude-Angle2/1
  Fourier1/2 -> Magnitude-Angle to Complex1/2
  Complex to Magnitude-Angle2/1 -> LPF1/1
  iq/1 -> Fourier1/1
  Constant1/1 -> Divide1/2
  LPF1/1 -> iq_sso_mag/1
  Fourier1/1 -> Magnitude-Angle to Complex1/1
  Complex to Magnitude-Angle2/2 -> Terminator1/1
  Magnitude-Angle to Complex1/1 -> Divide1/1
